simulink model "pid_gir_forskjellige"  (R2023b)
settings: Solver=VariableStepAuto  StartTime=0.0  StopTime=10  RelTol=1e-6
values from neighbouring files (symbols this model uses):
  bidrag_gir_front = 2*0.000327511    (= 0.000655022)    [modell_koeff.m]
  bidrag_gir_side = 0.00202665    [modell_koeff.m]
  Cd_front = 1.261    [modell_koeff.m]
  Cd_side = 1.410    (= 1.41)    [modell_koeff.m]
  g = 9.81    [modell_koeff.m]
  r_motor_gir = 0.3144    [modell_koeff.m]
  tetthet_vann = 1000    [modell_koeff.m]
  theta_motor_gir = deg2rad(90-79.7)    [modell_koeff.m]
  treghetsmoment_gir = 0.869830    (= 0.86983)    [modell_koeff.m]
libraries: simulink_extras x17, spsFirstOrderFilterLib x4, slpidlib x1
settings Model: Creator=kristianbirkeland  LastModifiedBy=bmm1
settings SolverCC: ZeroCrossAlgorithm=Adaptive
settings DebuggingCC: IgnoredZcDiagnostic=none  UnconnectedInputMsg=warning  UnconnectedOutputMsg=warning  UnconnectedLineMsg=warning
settings ModelReferenceCC: EnableRefExpFcnMdlSchedulingChecks=on
settings RTWCC: DLArmComputeVersion=19.05

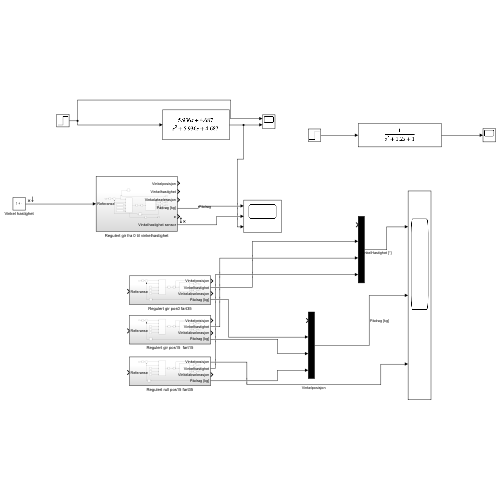
[thumbnail: Simulink's stored preview of the top-level diagram]
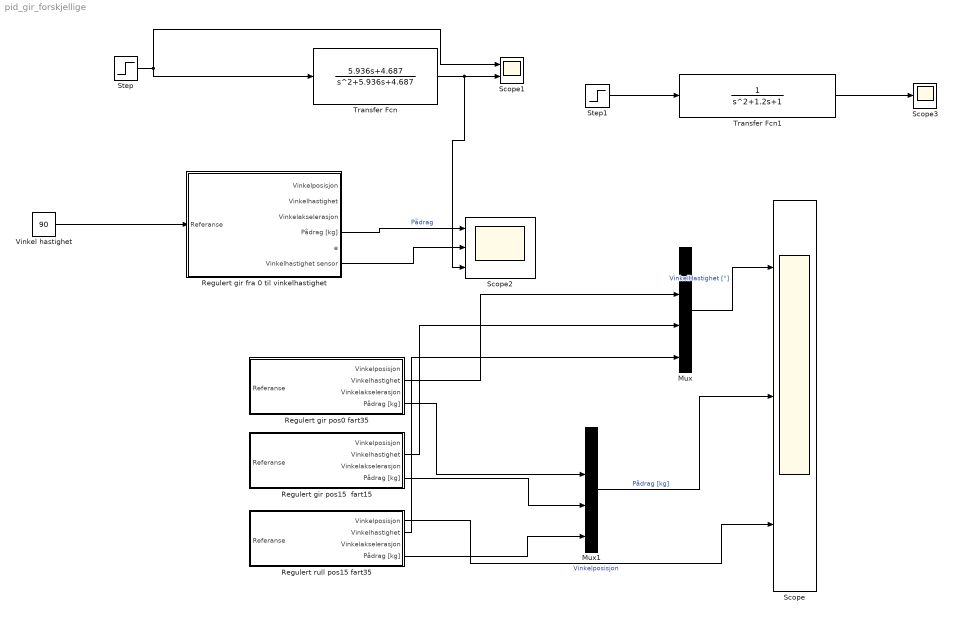
== system pid_gir_forskjellige ==
  Mux : Mux
  Mux1 : Mux
  Regulert gir fra 0 til vinkelhastighet : Subsystem
  Regulert gir pos0 fart35 : Subsystem
  Regulert gir pos15  fart15 : Subsystem
  Regulert rull pos15 fart35 : Subsystem
  Scope : Scope  NumInputPorts=3
  Scope1 : Scope  NumInputPorts=2
  Scope2 : Scope  NumInputPorts=3
  Scope3 : Scope
  Step : Step  Time=0  After=90  SampleTime=0
  Step1 : Step  After=90  SampleTime=0
  Transfer Fcn : TransferFcn  Numerator=[5.936 4.687]  Denominator=[1 5.936 4.687]
  Transfer Fcn1 : TransferFcn  Denominator=[1 1.2 1]
  Vinkel hastighet : Constant  Value=90
  wires:
  Vinkel hastighet/1 -> Regulert gir fra 0 til vinkelhastighet/1(Referanse)
  Regulert gir pos0 fart35/4(Pådrag [kg]) -> Mux1/2
  Regulert gir pos15  fart15/4(Pådrag [kg]) -> Mux1/3
  Regulert rull pos15 fart35/4(Pådrag [kg]) -> Mux1/4
  Mux/1 -> Scope/1  "VinkelHastighet [°]"
  Mux1/1 -> Scope/2  "Pådrag [kg]"
  Regulert gir pos0 fart35/2(Vinkelhastighet) -> Mux/2
  Regulert gir pos15  fart15/2(Vinkelhastighet) -> Mux/3
  Regulert rull pos15 fart35/2(Vinkelhastighet) -> Mux/4
  Regulert rull pos15 fart35/1(Vinkelposisjon) -> Scope/3  "Vinkelposisjon"
  Regulert gir fra 0 til vinkelhastighet/4(Pådrag [kg]) -> Scope2/1  "Pådrag"
  Regulert gir fra 0 til vinkelhastighet/6(Vinkelhastighet sensor) -> Scope2/2
  Transfer Fcn/1 -> Scope2/3, Scope1/2
  Step/1 -> Scope1/1, Transfer Fcn/1
  Step1/1 -> Transfer Fcn1/1
  Transfer Fcn1/1 -> Scope3/1

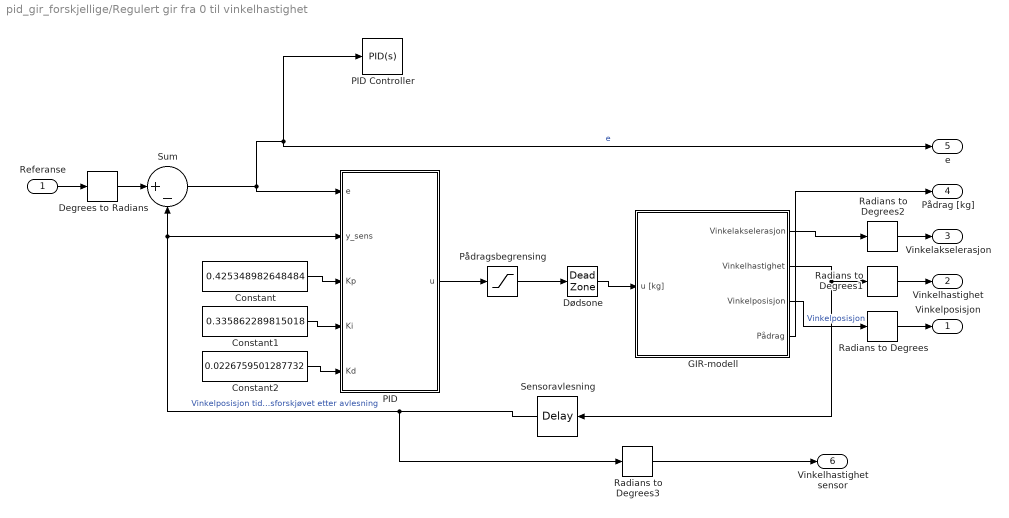
== system pid_gir_forskjellige/Regulert gir fra 0 til vinkelhastighet ==
  Referanse : Inport
  Constant : Constant  Value=0.425348982648484
  Constant1 : Constant  Value=0.335862289815018
  Constant2 : Constant  Value=0.0226759501287732
  Degrees to Radians : simulink_extras/Transformations/Degrees to Radians
  Dødsone : DeadZone  LowerValue=-0.05  UpperValue=0.05
  GIR-modell : Subsystem
  PID : Subsystem
  PID Controller : slpidlib/PID Controller  Controller=PID  Form=Parallel  TimeDomain=Continuous-time  UseExternalTs=off  SampleTime=-1  IntegratorMethod=Forward Euler  FilterMethod=Forward Euler  ControllerParametersSource=internal  P=0.425348982648484  I=0.335862289815018  UseKiTs=off  D=0.0226759501287732  N=546.991859681686  UseFilter=on  TunerSelectOption=Transfer Function Based (PID Tuner App)  InitialConditionSource=internal  InitialConditionForIntegrator=0  InitialConditionForFilter=0  DifferentiatorICPrevScaledInput=0  ExternalReset=none  TrackingMode=off  Kt=1  LimitOutput=off  SatLimitsSource=internal  UpperSaturationLimit=inf  LowerSaturationLimit=-inf  LinearizeAsGain=on  AntiWindupMode=none  Kb=1  LimitIntegrator=off  UpperIntegratorSaturationLimit=inf  LowerIntegratorSaturationLimit=-inf  POutMin=[]  POutMax=[]  IOutMin=[]  IOutMax=[]  DOutMin=[]  DOutMax=[]  NOutMin=[]  NOutMax=[]  SumOutMin=[]  SumOutMax=[]  SaturationOutMin=[]  SaturationOutMax=[]  PParamMin=[]  PParamMax=[]  IParamMin=[]  IParamMax=[]  DParamMin=[]  DParamMax=[]  NParamMin=[]  NParamMax=[]  KbParamMin=[]  KbParamMax=[]  KtParamMin=[]  KtParamMax=[]  KbOutMin=[]  KbOutMax=[]  KtOutMin=[]  KtOutMax=[]  IntegratorOutMin=[]  IntegratorOutMax=[]  FilterOutMin=[]  FilterOutMax=[]  SumI1OutMin=[]  SumI1OutMax=[]  SumI2OutMin=[]  SumI2OutMax=[]  SumI3OutMin=[]  SumI3OutMax=[]  SumI4OutMin=[]  SumI4OutMax=[]  SumDOutMin=[]  SumDOutMax=[]  DifferentiatorOutMin=[]  DifferentiatorOutMax=[]  FilterDiffOutCoefMin=[]  FilterDiffOutCoefMax=[]  ReciprocalOutMin=[]  ReciprocalOutMax=[]  SumDenOutMin=[]  SumDenOutMax=[]  SumNumOutMin=[]  SumNumOutMax=[]  DivideOutMin=[]  DivideOutMax=[]  UdiffTsProdOutMin=[]  UdiffTsProdOutMax=[]  NTsProdOutMin=[]  NTsProdOutMax=[]  UintegralTsProdOutMin=[]  UintegralTsProdOutMax=[]  UngainTsProdOutMin=[]  UngainTsProdOutMax=[]  ClampingZeroOutDataTypeStr=Inherit: Inherit via back propagation  ClampingZeroOutMin=[]  ClampingZeroOutMax=[]  FilterDenConstantOutDataTypeStr=Inherit: Inherit via back propagation  FilterDenConstantOutMin=[]  FilterDenConstantOutMax=[]  PCopyOutDataTypeStr=Inherit: Inherit via back propagation  PCopyOutMin=[]  PCopyOutMax=[]  NCopyOutDataTypeStr=Inherit: Inherit via back propagation  NCopyOutMin=[]  NCopyOutMax=[]  IntegratorContinuousStateAttributes=''  IntegratorStateMustResolveToSignalObject=off  IntegratorRTWStateStorageClass=Auto  FilterContinuousStateAttributes=''  FilterStateMustResolveToSignalObject=off  FilterRTWStateStorageClass=Auto  ParallelPVariant=InternalParameters  IdealPVariant=Disabled  IVariant=InternalParameters  DVariant=InternalParameters  IntegratorVariant=Continuous  SatVariant=Disabled  AWVariant=Passthrough  PCopyVariant=Disabled  TRVariant=Disabled  FdbkBlocksVariant=Forward  IdealPFdbkVariant=Disabled  SatFdbkVariant=Disabled  DerivativeFilterVariant=ContFilter  NVariant=InternalParameters  NCopyVariant=Disabled  FilterICVariant=InternalICsFilter  IntegratorICVariant=InternalICs  ExternalResetVariant=Disabled  TRSumVariant=Passthrough  SumFdbkVariant=Disabled  SumVariant=Sum_PID  TsampFilterVariant=InternalTs  TsampNgainVariant=Passthrough  TsampIntegralVariant=Disabled_SignalSpec  ExternalSaturationOutDataTypeStr=Inherit: Same as second input
  Pådragsbegrensing : Saturate  UpperLimit=2.7  LowerLimit=-2.7
  Radians to Degrees{,1..3} (4 alike) : simulink_extras/Transformations/Radians to Degrees
  Sensoravlesning : TransportDelay  DelayTime=0.2
  Sum : Sum  Inputs=|+-
  Vinkelposisjon : Outport
  Vinkelhastighet : Outport  Port=2
  Vinkelakselerasjon : Outport  Port=3
  Pådrag [kg] : Outport  Port=4
  e : Outport  Port=5
  Vinkelhastighet sensor : Outport  Port=6
  wires:
  GIR-modell/2(" Vinkelhastighet") -> Sensoravlesning/1, Radians to Degrees1/1
  Constant1/1 -> PID/4(Ki)
  Constant/1 -> PID/3(Kp)
  Constant2/1 -> PID/5(Kd)
  Sum/1 -> PID Controller/1, e/1, PID/1(e)  "e"
  GIR-modell/3(Vinkelposisjon) -> Radians to Degrees/1  "Vinkelposisjon"
  Radians to Degrees/1 -> Vinkelposisjon/1
  Radians to Degrees1/1 -> Vinkelhastighet/1
  GIR-modell/1(" Vinkelakselerasjon") -> Radians to Degrees2/1
  Radians to Degrees2/1 -> Vinkelakselerasjon/1
  Referanse/1 -> Degrees to Radians/1
  Degrees to Radians/1 -> Sum/1
  Sensoravlesning/1 -> Radians to Degrees3/1, Sum/2, PID/2(y_sens)  "Vinkelposisjon tidsforskjøvet etter avlesning"
  Pådragsbegrensing/1 -> Dødsone/1
  Dødsone/1 -> GIR-modell/1(u [kg])
  GIR-modell/4(" Pådrag") -> Pådrag [kg]/1
  Radians to Degrees3/1 -> Vinkelhastighet sensor/1
  PID/1(u) -> Pådragsbegrensing/1

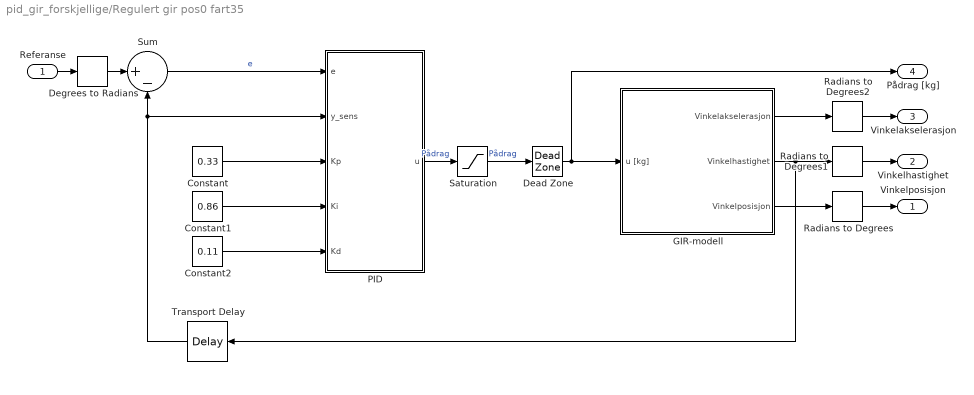
== system pid_gir_forskjellige/Regulert gir pos0 fart35 ==
  Referanse : Inport
  Constant : Constant  Value=0.33
  Constant1 : Constant  Value=0.86
  Constant2 : Constant  Value=0.11
  Dead Zone : DeadZone  LowerValue=-0.05  UpperValue=0.05
  Degrees to Radians : simulink_extras/Transformations/Degrees to Radians
  GIR-modell : Subsystem
  PID : Subsystem
  Radians to Degrees : simulink_extras/Transformations/Radians to Degrees
  Radians to Degrees1 : simulink_extras/Transformations/Radians to Degrees
  Radians to Degrees2 : simulink_extras/Transformations/Radians to Degrees
  Saturation : Saturate  UpperLimit=2.7  LowerLimit=-2.7
  Sum : Sum  Inputs=|+-
  Transport Delay : TransportDelay  DelayTime=0.2
  Vinkelposisjon : Outport
  Vinkelhastighet : Outport  Port=2
  Vinkelakselerasjon : Outport  Port=3
  Pådrag [kg] : Outport  Port=4
  wires:
  GIR-modell/2(" Vinkelhastighet") -> Transport Delay/1, Radians to Degrees1/1
  Constant1/1 -> PID/4(Ki)
  Constant/1 -> PID/3(Kp)
  Constant2/1 -> PID/5(Kd)
  Sum/1 -> PID/1(e)  "e"
  PID/1(u) -> Saturation/1  "Pådrag"
  Transport Delay/1 -> PID/2(y_sens), Sum/2
  GIR-modell/3(Vinkelposisjon) -> Radians to Degrees/1
  Saturation/1 -> Dead Zone/1  "Pådrag"
  Radians to Degrees/1 -> Vinkelposisjon/1
  Radians to Degrees1/1 -> Vinkelhastighet/1
  GIR-modell/1(" Vinkelakselerasjon") -> Radians to Degrees2/1
  Radians to Degrees2/1 -> Vinkelakselerasjon/1
  Referanse/1 -> Degrees to Radians/1
  Degrees to Radians/1 -> Sum/1
  Dead Zone/1 -> GIR-modell/1(u [kg]), Pådrag [kg]/1

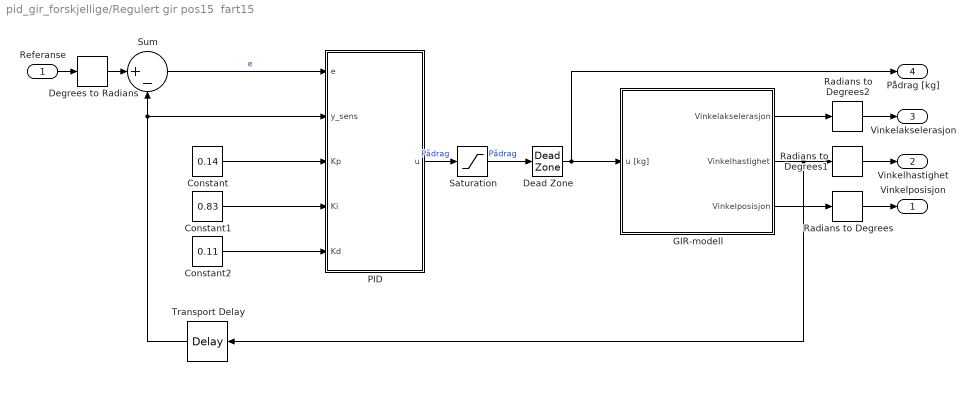
== system pid_gir_forskjellige/Regulert gir pos15  fart15 ==
  Referanse : Inport
  Constant : Constant  Value=0.14
  Constant1 : Constant  Value=0.83
  Constant2 : Constant  Value=0.11
  Dead Zone : DeadZone  LowerValue=-0.05  UpperValue=0.05
  Degrees to Radians : simulink_extras/Transformations/Degrees to Radians
  GIR-modell : Subsystem
  PID : Subsystem
  Radians to Degrees : simulink_extras/Transformations/Radians to Degrees
  Radians to Degrees1 : simulink_extras/Transformations/Radians to Degrees
  Radians to Degrees2 : simulink_extras/Transformations/Radians to Degrees
  Saturation : Saturate  UpperLimit=2.7  LowerLimit=-2.7
  Sum : Sum  Inputs=|+-
  Transport Delay : TransportDelay  DelayTime=0.2
  Vinkelposisjon : Outport
  Vinkelhastighet : Outport  Port=2
  Vinkelakselerasjon : Outport  Port=3
  Pådrag [kg] : Outport  Port=4
  wires:
  GIR-modell/2(" Vinkelhastighet") -> Transport Delay/1, Radians to Degrees1/1
  Constant1/1 -> PID/4(Ki)
  Constant/1 -> PID/3(Kp)
  Constant2/1 -> PID/5(Kd)
  Sum/1 -> PID/1(e)  "e"
  PID/1(u) -> Saturation/1  "Pådrag"
  Transport Delay/1 -> PID/2(y_sens), Sum/2
  GIR-modell/3(Vinkelposisjon) -> Radians to Degrees/1
  Saturation/1 -> Dead Zone/1  "Pådrag"
  Radians to Degrees/1 -> Vinkelposisjon/1
  Radians to Degrees1/1 -> Vinkelhastighet/1
  GIR-modell/1(" Vinkelakselerasjon") -> Radians to Degrees2/1
  Radians to Degrees2/1 -> Vinkelakselerasjon/1
  Referanse/1 -> Degrees to Radians/1
  Degrees to Radians/1 -> Sum/1
  Dead Zone/1 -> GIR-modell/1(u [kg]), Pådrag [kg]/1

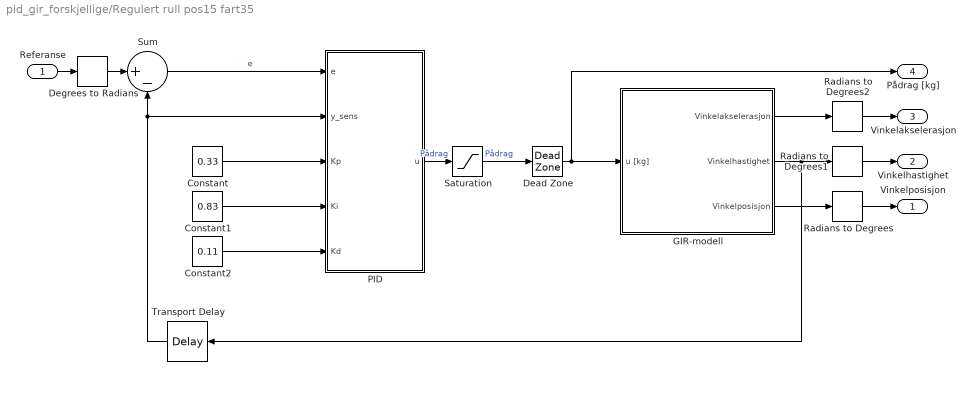
== system pid_gir_forskjellige/Regulert rull pos15 fart35 ==
  Referanse : Inport
  Constant : Constant  Value=0.33
  Constant1 : Constant  Value=0.83
  Constant2 : Constant  Value=0.11
  Dead Zone : DeadZone  LowerValue=-0.05  UpperValue=0.05
  Degrees to Radians : simulink_extras/Transformations/Degrees to Radians
  GIR-modell : Subsystem
  PID : Subsystem
  Radians to Degrees : simulink_extras/Transformations/Radians to Degrees
  Radians to Degrees1 : simulink_extras/Transformations/Radians to Degrees
  Radians to Degrees2 : simulink_extras/Transformations/Radians to Degrees
  Saturation : Saturate  UpperLimit=2.7  LowerLimit=-2.7
  Sum : Sum  Inputs=|+-
  Transport Delay : TransportDelay  DelayTime=0.2
  Vinkelposisjon : Outport
  Vinkelhastighet : Outport  Port=2
  Vinkelakselerasjon : Outport  Port=3
  Pådrag [kg] : Outport  Port=4
  wires:
  GIR-modell/2(" Vinkelhastighet") -> Transport Delay/1, Radians to Degrees1/1
  Constant1/1 -> PID/4(Ki)
  Constant/1 -> PID/3(Kp)
  Constant2/1 -> PID/5(Kd)
  Sum/1 -> PID/1(e)  "e"
  PID/1(u) -> Saturation/1  "Pådrag"
  Transport Delay/1 -> PID/2(y_sens), Sum/2
  GIR-modell/3(Vinkelposisjon) -> Radians to Degrees/1
  Saturation/1 -> Dead Zone/1  "Pådrag"
  Radians to Degrees/1 -> Vinkelposisjon/1
  Radians to Degrees1/1 -> Vinkelhastighet/1
  GIR-modell/1(" Vinkelakselerasjon") -> Radians to Degrees2/1
  Radians to Degrees2/1 -> Vinkelakselerasjon/1
  Referanse/1 -> Degrees to Radians/1
  Degrees to Radians/1 -> Sum/1
  Dead Zone/1 -> GIR-modell/1(u [kg]), Pådrag [kg]/1

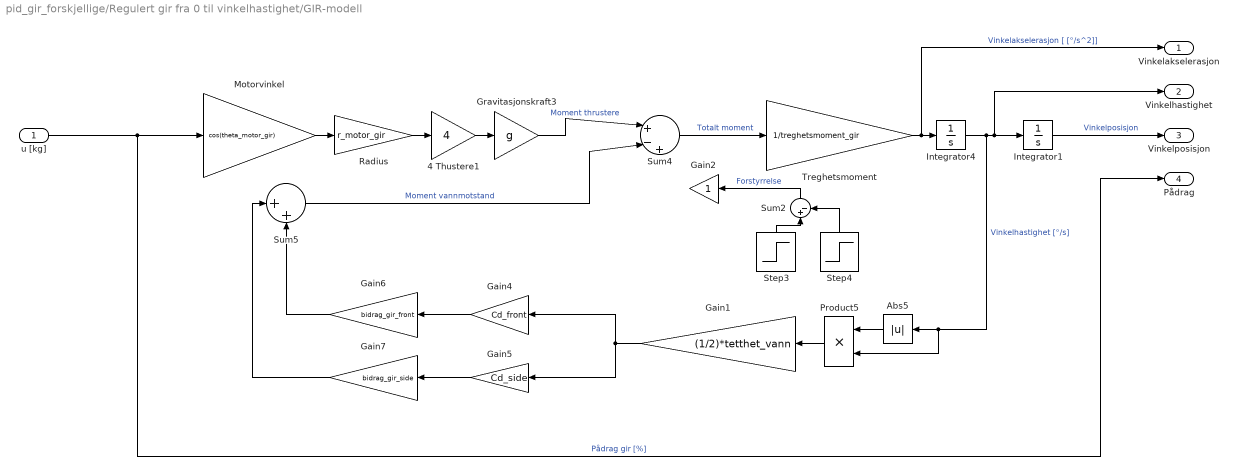
== system pid_gir_forskjellige/Regulert gir fra 0 til vinkelhastighet/GIR-modell ==
  u [kg] : Inport
  4 Thustere1 : Gain  Gain=4
  Abs5 : Abs  SaturateOnIntegerOverflow=off
  Gain1 : Gain  Gain=(1/2)*tetthet_vann
  Gain2 : Gain
  Gain4 : Gain  Gain=Cd_front
  Gain5 : Gain  Gain=Cd_side
  Gain6 : Gain  Gain=bidrag_gir_front
  Gain7 : Gain  Gain=bidrag_gir_side
  Gravitasjonskraft3 : Gain  Gain=g
  Integrator1 : Integrator
  Integrator4 : Integrator
  Motorvinkel : Gain  Gain=cos(theta_motor_gir)
  Product5 : Product
  Radius : Gain  Gain=r_motor_gir
  Step3 : Step  Time=10  After=5  SampleTime=0
  Step4 : Step  Time=25  After=5  SampleTime=0
  Sum2 : Sum  Inputs=|+-
  Sum4 : Sum  Inputs=|+-+
  Sum5 : Sum  Inputs=|++
  Treghetsmoment : Gain  Gain=1/treghetsmoment_gir
  " Vinkelakselerasjon" : Outport
  " Vinkelhastighet" : Outport  Port=2
  Vinkelposisjon : Outport  Port=3
  " Pådrag" : Outport  Port=4
  wires:
  Gain4/1 -> Gain6/1
  Radius/1 -> 4 Thustere1/1
  Sum4/1 -> Treghetsmoment/1  "Totalt moment"
  Abs5/1 -> Product5/1
  Product5/1 -> Gain1/1
  Sum5/1 -> Sum4/2  "Moment vannmotstand"
  Gain6/1 -> Sum5/2
  Gain7/1 -> Sum5/1
  Gravitasjonskraft3/1 -> Sum4/1  "Moment thrustere"
  Gain1/1 -> Gain5/1, Gain4/1
  Gain5/1 -> Gain7/1
  u [kg]/1 -> " Pådrag"/1, Motorvinkel/1  "Pådrag gir [%]"
  Motorvinkel/1 -> Radius/1
  Integrator4/1 -> " Vinkelhastighet"/1, Integrator1/1, Abs5/1, Product5/2  "Vinkelhastighet [°/s]"
  4 Thustere1/1 -> Gravitasjonskraft3/1
  Treghetsmoment/1 -> " Vinkelakselerasjon"/1, Integrator4/1  "Vinkelakselerasjon [ [°/s^2]]"
  Sum2/1 -> Gain2/1  "Forstyrrelse"
  Step4/1 -> Sum2/2
  Step3/1 -> Sum2/1
  Integrator1/1 -> Vinkelposisjon/1  "Vinkelposisjon"

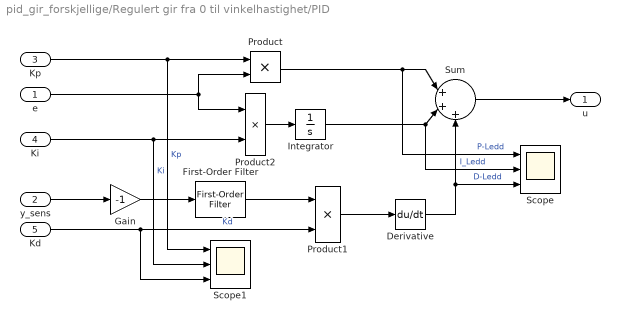
== system pid_gir_forskjellige/Regulert gir fra 0 til vinkelhastighet/PID ==
  e : Inport
  y_sens : Inport  Port=2
  Kp : Inport  Port=3
  Ki : Inport  Port=4
  Kd : Inport  Port=5
  Derivative : Derivative
  First-Order Filter : spsFirstOrderFilterLib/First-Order Filter  FilterType=Lowpass  Tc=(0.11/0.14)*0.05  Ts=0  Initialize=on  Vac_Init=[0, 0, 60]  Vdc_Init=0  PlotResponse=off  FreqRange="[0,  200,  1]"
  Gain : Gain  Gain=-1
  Integrator : Integrator  LimitOutput=on
  Product : Product
  Product1 : Product
  Product2 : Product
  Scope : Scope  NumInputPorts=3
  Scope1 : Scope  NumInputPorts=3
  Sum : Sum  Inputs=|+++
  u : Outport
  wires:
  e/1 -> Product2/1, Product/2
  Sum/1 -> u/1
  y_sens/1 -> Gain/1
  Kd/1 -> Scope1/3, Product1/2  "Kd"
  Ki/1 -> Scope1/2, Product2/2  "Ki"
  Product2/1 -> Integrator/1
  Product1/1 -> Derivative/1
  Derivative/1 -> Sum/3, Scope/3  "D-Ledd"
  Product/1 -> Scope/1, Sum/1  "P-Ledd"
  Integrator/1 -> Sum/2, Scope/2  "I_Ledd"
  Kp/1 -> Scope1/1, Product/1  "Kp"
  Gain/1 -> First-Order Filter/1
  First-Order Filter/1 -> Product1/1

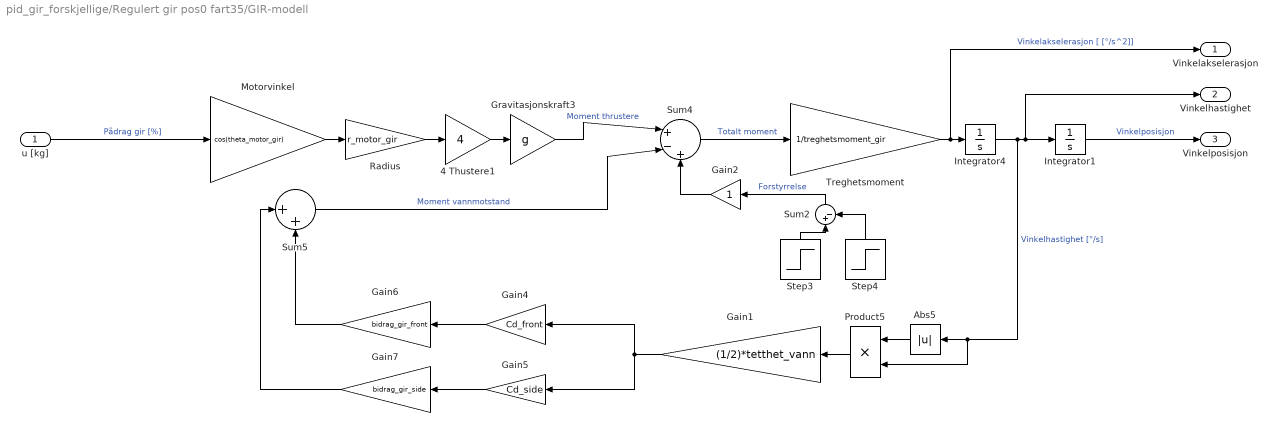
== system pid_gir_forskjellige/Regulert gir pos0 fart35/GIR-modell ==
  u [kg] : Inport
  4 Thustere1 : Gain  Gain=4
  Abs5 : Abs  SaturateOnIntegerOverflow=off
  Gain1 : Gain  Gain=(1/2)*tetthet_vann
  Gain2 : Gain
  Gain4 : Gain  Gain=Cd_front
  Gain5 : Gain  Gain=Cd_side
  Gain6 : Gain  Gain=bidrag_gir_front
  Gain7 : Gain  Gain=bidrag_gir_side
  Gravitasjonskraft3 : Gain  Gain=g
  Integrator1 : Integrator  InitialCondition=pi/4
  Integrator4 : Integrator
  Motorvinkel : Gain  Gain=cos(theta_motor_gir)
  Product5 : Product
  Radius : Gain  Gain=r_motor_gir
  Step3 : Step  Time=10  After=5  SampleTime=0
  Step4 : Step  Time=25  After=5  SampleTime=0
  Sum2 : Sum  Inputs=|+-
  Sum4 : Sum  Inputs=|+-+
  Sum5 : Sum  Inputs=|++
  Treghetsmoment : Gain  Gain=1/treghetsmoment_gir
  " Vinkelakselerasjon" : Outport
  " Vinkelhastighet" : Outport  Port=2
  Vinkelposisjon : Outport  Port=3
  wires:
  Gain4/1 -> Gain6/1
  Radius/1 -> 4 Thustere1/1
  Sum4/1 -> Treghetsmoment/1  "Totalt moment"
  Abs5/1 -> Product5/1
  Product5/1 -> Gain1/1
  Sum5/1 -> Sum4/2  "Moment vannmotstand"
  Gain6/1 -> Sum5/2
  Gain7/1 -> Sum5/1
  Gravitasjonskraft3/1 -> Sum4/1  "Moment thrustere"
  Gain1/1 -> Gain5/1, Gain4/1
  Gain5/1 -> Gain7/1
  u [kg]/1 -> Motorvinkel/1  "Pådrag gir [%]"
  Motorvinkel/1 -> Radius/1
  Integrator4/1 -> " Vinkelhastighet"/1, Integrator1/1, Abs5/1, Product5/2  "Vinkelhastighet [°/s]"
  4 Thustere1/1 -> Gravitasjonskraft3/1
  Treghetsmoment/1 -> " Vinkelakselerasjon"/1, Integrator4/1  "Vinkelakselerasjon [ [°/s^2]]"
  Sum2/1 -> Gain2/1  "Forstyrrelse"
  Gain2/1 -> Sum4/3
  Step4/1 -> Sum2/2
  Step3/1 -> Sum2/1
  Integrator1/1 -> Vinkelposisjon/1  "Vinkelposisjon"

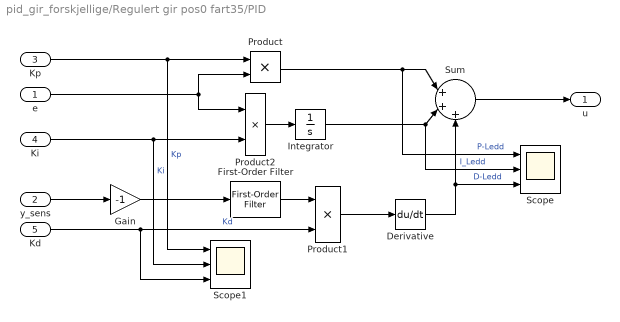
== system pid_gir_forskjellige/Regulert gir pos0 fart35/PID ==
  e : Inport
  y_sens : Inport  Port=2
  Kp : Inport  Port=3
  Ki : Inport  Port=4
  Kd : Inport  Port=5
  Derivative : Derivative
  First-Order Filter : spsFirstOrderFilterLib/First-Order Filter  FilterType=Lowpass  Tc=(0.11/0.33)*0.05  Ts=0  Initialize=on  Vac_Init=[0, 0, 60]  Vdc_Init=0  PlotResponse=off  FreqRange="[0,  200,  1]"
  Gain : Gain  Gain=-1
  Integrator : Integrator  LimitOutput=on  UpperSaturationLimit=0.5  LowerSaturationLimit=-2
  Product : Product
  Product1 : Product
  Product2 : Product
  Scope : Scope  NumInputPorts=3
  Scope1 : Scope  NumInputPorts=3
  Sum : Sum  Inputs=|+++
  u : Outport
  wires:
  e/1 -> Product2/1, Product/2
  Sum/1 -> u/1
  y_sens/1 -> Gain/1
  First-Order Filter/1 -> Product1/1
  Kd/1 -> Scope1/3, Product1/2  "Kd"
  Ki/1 -> Scope1/2, Product2/2  "Ki"
  Product2/1 -> Integrator/1
  Product1/1 -> Derivative/1
  Derivative/1 -> Sum/3, Scope/3  "D-Ledd"
  Gain/1 -> First-Order Filter/1
  Product/1 -> Scope/1, Sum/1  "P-Ledd"
  Integrator/1 -> Sum/2, Scope/2  "I_Ledd"
  Kp/1 -> Scope1/1, Product/1  "Kp"

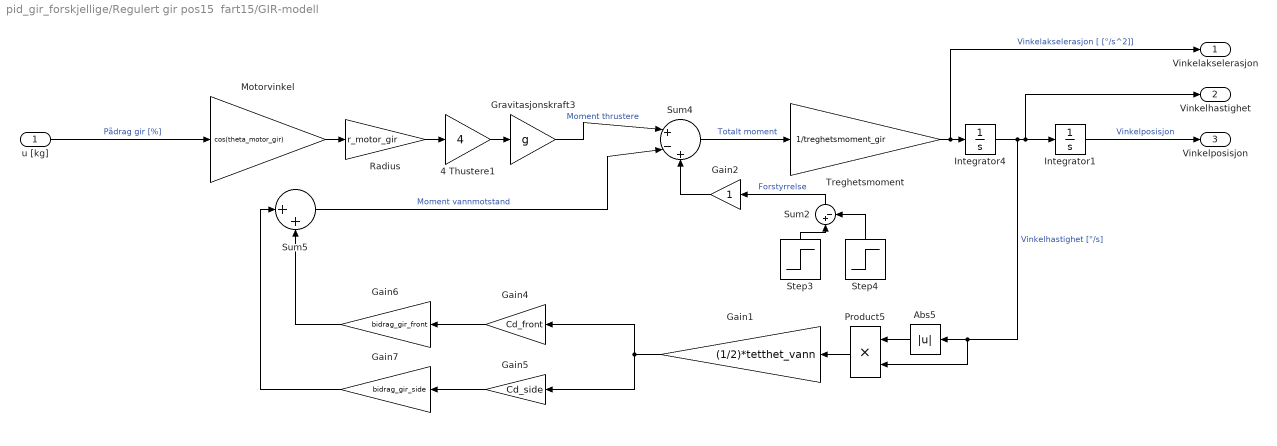
== system pid_gir_forskjellige/Regulert gir pos15  fart15/GIR-modell ==
  u [kg] : Inport
  4 Thustere1 : Gain  Gain=4
  Abs5 : Abs  SaturateOnIntegerOverflow=off
  Gain1 : Gain  Gain=(1/2)*tetthet_vann
  Gain2 : Gain
  Gain4 : Gain  Gain=Cd_front
  Gain5 : Gain  Gain=Cd_side
  Gain6 : Gain  Gain=bidrag_gir_front
  Gain7 : Gain  Gain=bidrag_gir_side
  Gravitasjonskraft3 : Gain  Gain=g
  Integrator1 : Integrator  InitialCondition=pi/4
  Integrator4 : Integrator
  Motorvinkel : Gain  Gain=cos(theta_motor_gir)
  Product5 : Product
  Radius : Gain  Gain=r_motor_gir
  Step3 : Step  Time=10  After=5  SampleTime=0
  Step4 : Step  Time=25  After=5  SampleTime=0
  Sum2 : Sum  Inputs=|+-
  Sum4 : Sum  Inputs=|+-+
  Sum5 : Sum  Inputs=|++
  Treghetsmoment : Gain  Gain=1/treghetsmoment_gir
  " Vinkelakselerasjon" : Outport
  " Vinkelhastighet" : Outport  Port=2
  Vinkelposisjon : Outport  Port=3
  wires:
  Gain4/1 -> Gain6/1
  Radius/1 -> 4 Thustere1/1
  Sum4/1 -> Treghetsmoment/1  "Totalt moment"
  Abs5/1 -> Product5/1
  Product5/1 -> Gain1/1
  Sum5/1 -> Sum4/2  "Moment vannmotstand"
  Gain6/1 -> Sum5/2
  Gain7/1 -> Sum5/1
  Gravitasjonskraft3/1 -> Sum4/1  "Moment thrustere"
  Gain1/1 -> Gain5/1, Gain4/1
  Gain5/1 -> Gain7/1
  u [kg]/1 -> Motorvinkel/1  "Pådrag gir [%]"
  Motorvinkel/1 -> Radius/1
  Integrator4/1 -> " Vinkelhastighet"/1, Integrator1/1, Abs5/1, Product5/2  "Vinkelhastighet [°/s]"
  4 Thustere1/1 -> Gravitasjonskraft3/1
  Treghetsmoment/1 -> " Vinkelakselerasjon"/1, Integrator4/1  "Vinkelakselerasjon [ [°/s^2]]"
  Sum2/1 -> Gain2/1  "Forstyrrelse"
  Gain2/1 -> Sum4/3
  Step4/1 -> Sum2/2
  Step3/1 -> Sum2/1
  Integrator1/1 -> Vinkelposisjon/1  "Vinkelposisjon"

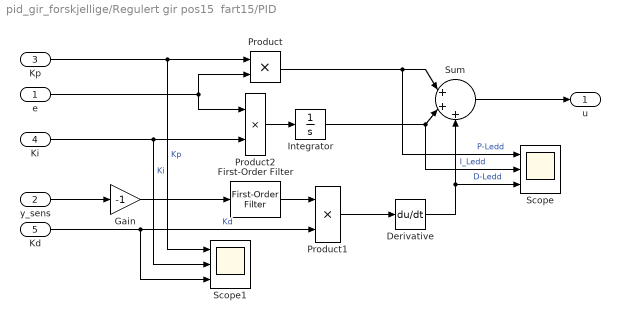
== system pid_gir_forskjellige/Regulert gir pos15  fart15/PID ==
  e : Inport
  y_sens : Inport  Port=2
  Kp : Inport  Port=3
  Ki : Inport  Port=4
  Kd : Inport  Port=5
  Derivative : Derivative
  First-Order Filter : spsFirstOrderFilterLib/First-Order Filter  FilterType=Lowpass  Tc=(0.11/0.14)*0.05  Ts=0  Initialize=on  Vac_Init=[0, 0, 60]  Vdc_Init=0  PlotResponse=off  FreqRange="[0,  200,  1]"
  Gain : Gain  Gain=-1
  Integrator : Integrator  LimitOutput=on  UpperSaturationLimit=0.5  LowerSaturationLimit=-2
  Product : Product
  Product1 : Product
  Product2 : Product
  Scope : Scope  NumInputPorts=3
  Scope1 : Scope  NumInputPorts=3
  Sum : Sum  Inputs=|+++
  u : Outport
  wires:
  e/1 -> Product2/1, Product/2
  Sum/1 -> u/1
  y_sens/1 -> Gain/1
  First-Order Filter/1 -> Product1/1
  Kd/1 -> Scope1/3, Product1/2  "Kd"
  Ki/1 -> Scope1/2, Product2/2  "Ki"
  Product2/1 -> Integrator/1
  Product1/1 -> Derivative/1
  Derivative/1 -> Sum/3, Scope/3  "D-Ledd"
  Gain/1 -> First-Order Filter/1
  Product/1 -> Scope/1, Sum/1  "P-Ledd"
  Integrator/1 -> Sum/2, Scope/2  "I_Ledd"
  Kp/1 -> Scope1/1, Product/1  "Kp"

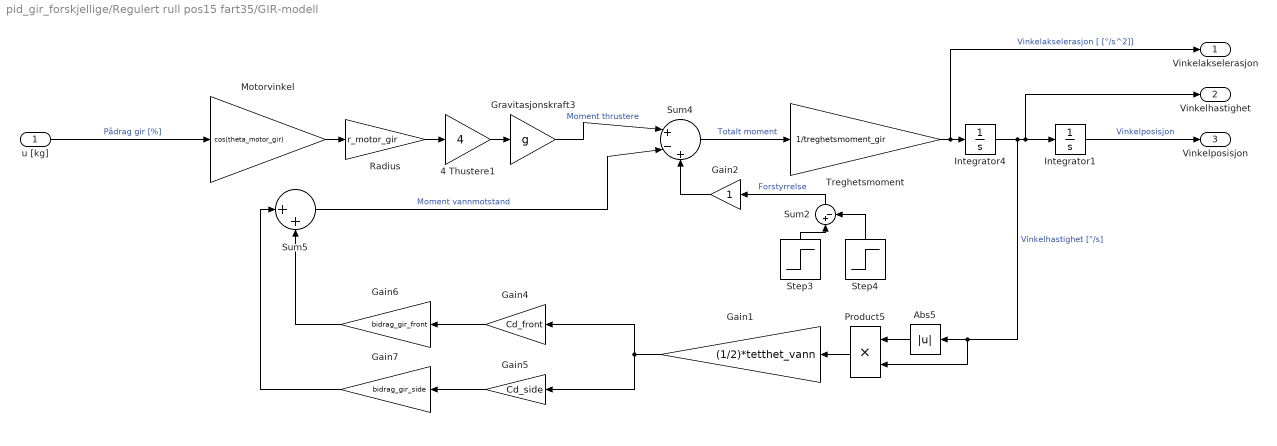
== system pid_gir_forskjellige/Regulert rull pos15 fart35/GIR-modell ==
  u [kg] : Inport
  4 Thustere1 : Gain  Gain=4
  Abs5 : Abs  SaturateOnIntegerOverflow=off
  Gain1 : Gain  Gain=(1/2)*tetthet_vann
  Gain2 : Gain
  Gain4 : Gain  Gain=Cd_front
  Gain5 : Gain  Gain=Cd_side
  Gain6 : Gain  Gain=bidrag_gir_front
  Gain7 : Gain  Gain=bidrag_gir_side
  Gravitasjonskraft3 : Gain  Gain=g
  Integrator1 : Integrator  InitialCondition=pi/4
  Integrator4 : Integrator
  Motorvinkel : Gain  Gain=cos(theta_motor_gir)
  Product5 : Product
  Radius : Gain  Gain=r_motor_gir
  Step3 : Step  Time=10  After=5  SampleTime=0
  Step4 : Step  Time=25  After=5  SampleTime=0
  Sum2 : Sum  Inputs=|+-
  Sum4 : Sum  Inputs=|+-+
  Sum5 : Sum  Inputs=|++
  Treghetsmoment : Gain  Gain=1/treghetsmoment_gir
  " Vinkelakselerasjon" : Outport
  " Vinkelhastighet" : Outport  Port=2
  Vinkelposisjon : Outport  Port=3
  wires:
  Gain4/1 -> Gain6/1
  Radius/1 -> 4 Thustere1/1
  Sum4/1 -> Treghetsmoment/1  "Totalt moment"
  Abs5/1 -> Product5/1
  Product5/1 -> Gain1/1
  Sum5/1 -> Sum4/2  "Moment vannmotstand"
  Gain6/1 -> Sum5/2
  Gain7/1 -> Sum5/1
  Gravitasjonskraft3/1 -> Sum4/1  "Moment thrustere"
  Gain1/1 -> Gain5/1, Gain4/1
  Gain5/1 -> Gain7/1
  u [kg]/1 -> Motorvinkel/1  "Pådrag gir [%]"
  Motorvinkel/1 -> Radius/1
  Integrator4/1 -> " Vinkelhastighet"/1, Integrator1/1, Abs5/1, Product5/2  "Vinkelhastighet [°/s]"
  4 Thustere1/1 -> Gravitasjonskraft3/1
  Treghetsmoment/1 -> " Vinkelakselerasjon"/1, Integrator4/1  "Vinkelakselerasjon [ [°/s^2]]"
  Sum2/1 -> Gain2/1  "Forstyrrelse"
  Gain2/1 -> Sum4/3
  Step4/1 -> Sum2/2
  Step3/1 -> Sum2/1
  Integrator1/1 -> Vinkelposisjon/1  "Vinkelposisjon"

== system pid_gir_forskjellige/Regulert rull pos15 fart35/PID ==
  e : Inport
  y_sens : Inport  Port=2
  Kp : Inport  Port=3
  Ki : Inport  Port=4
  Kd : Inport  Port=5
  Derivative : Derivative
  First-Order Filter : spsFirstOrderFilterLib/First-Order Filter  FilterType=Lowpass  Tc=(0.11/0.33)*0.05  Ts=0  Initialize=on  Vac_Init=[0, 0, 60]  Vdc_Init=0  PlotResponse=off  FreqRange="[0,  200,  1]"
  Gain : Gain  Gain=-1
  Integrator : Integrator  LimitOutput=on  UpperSaturationLimit=0.5  LowerSaturationLimit=-2
  Product : Product
  Product1 : Product
  Product2 : Product
  Scope : Scope  NumInputPorts=3
  Scope1 : Scope  NumInputPorts=3
  Sum : Sum  Inputs=|+++
  u : Outport
  wires:
  e/1 -> Product2/1, Product/2
  Sum/1 -> u/1
  y_sens/1 -> Gain/1
  First-Order Filter/1 -> Product1/1
  Kd/1 -> Scope1/3, Product1/2  "Kd"
  Ki/1 -> Scope1/2, Product2/2  "Ki"
  Product2/1 -> Integrator/1
  Product1/1 -> Derivative/1
  Derivative/1 -> Sum/3, Scope/3  "D-Ledd"
  Gain/1 -> First-Order Filter/1
  Product/1 -> Scope/1, Sum/1  "P-Ledd"
  Integrator/1 -> Sum/2, Scope/2  "I_Ledd"
  Kp/1 -> Scope1/1, Product/1  "Kp"
